simulink model "representacionabloquess"  (R2025a)
settings: Solver=ode45  StartTime=0.0  StopTime=10.0  RelTol=1e-3

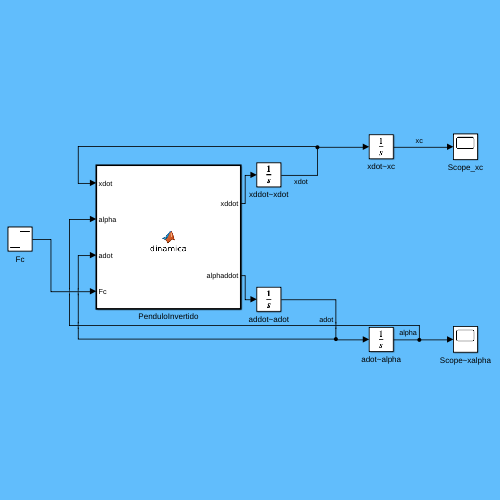
[thumbnail: Simulink's stored preview of the top-level diagram]
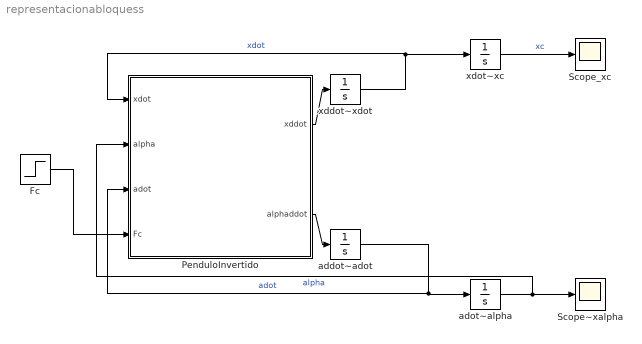
== system representacionabloquess ==
  Fc : Step  Time=0  After=0  SampleTime=0
  PenduloInvertido : MATLAB Function  TreatAsAtomicUnit=on
  Scope_xc : Scope
      settings: ActiveDisplayYMinimum=-31.977390230636651  ActiveDisplayYMaximum=46.328440296224436
  Scope~xalpha : Scope
      settings: ActiveDisplayYMinimum=-115.40515409428737  ActiveDisplayYMaximum=252.16601481498984
  addot~adot : Integrator
  adot~alpha : Integrator  InitialCondition=pi/180  AbsoluteTolerance=1
  xddot~xdot : Integrator
  xdot~xc : Integrator
  wires:
  xddot~xdot/1 -> xdot~xc/1, PenduloInvertido/1(xdot)  "xdot"
  xdot~xc/1 -> Scope_xc/1  "xc"
  addot~adot/1 -> PenduloInvertido/3(adot), adot~alpha/1  "adot"
  adot~alpha/1 -> PenduloInvertido/2(alpha), Scope~xalpha/1  "alpha"
  PenduloInvertido/1(xddot) -> xddot~xdot/1
  PenduloInvertido/2(alphaddot) -> addot~adot/1
  Fc/1 -> PenduloInvertido/4(Fc)

== matlab function representacionabloquess/PenduloInvertido ==
  data: xdot input; alpha input; adot input; xddot output; alphaddot output; Fc input
function [xddot, alphaddot] = dinamica(xdot, alpha, adot, Fc)
Ip  = 0.0079;     % kg*m^
Mc  = 0.7031;     % kg
lp  = 0.3302;     % m
Mp  = 0.23;       % kg
Beq = 4.3;        % N*s/m
g   = 9.81;       % m/s^2
Bp  = 0.0024;     % N*m*s/rad

D = (Mc+Mp)*Ip + Mc*Mp*lp^2 + (Mp^2*lp^2)*(sin(alpha)^2);

Nx = (Ip + Mp*lp^2)*Fc ...
     + (Mp^2*lp^2*g)*cos(alpha)*sin(alpha) ...
     - (Ip + Mp*lp^2)*Beq*xdot ...
     - (Ip*Mp*lp - Mp^2*lp^3)*(adot^2)*sin(alpha) ...
     - (Mp*lp*Bp)*adot*cos(alpha);

Na = ((Mc+Mp)*Mp*g*lp)*sin(alpha) ...
     - ((Mc+Mp)*Bp)*adot ...
     + (Fc*Mp*lp)*cos(alpha) ...
     - (Mp^2*lp^2)*(adot^2)*sin(alpha)*cos(alpha) ...
     - (Beq*Mp*lp)*xdot*cos(alpha);

xddot = Nx / D;
alphaddot = Na / D;
end
